simulink model "hw_interface_uart_data_sender"  (R2023b)
settings: Solver=FixedStepAuto  StartTime=0.0  StopTime=inf  FixedStep=0.001  RelTol=1e-3  EnableMultiTasking=on
undefined symbols (not defined in the file): LF
libraries: embeddedblockslib x1, mbedblockslib x1
settings Model: SimulationMode=external  ExtModeEnableFloating=off  ExtModeTrigDuration=10  Creator=kiraa  LastModifiedBy=kiraa
settings DataIOCC: SaveOutput=off  DSMLogging=off  SaveTime=off  TimeSaveName=time
settings OptimizationCC: StrengthReduction=on  PassReuseOutputArgsAs=Individual arguments  ZeroExternalMemoryAtStartup=off  ZeroInternalMemoryAtStartup=off  MaxStackSize=64  OptimizeBlockOrder=speed  OptimizationPriority=Speed  OptimizationCustomize=off  MultiThreadedLoops=on  EfficientTunableParamExpr=on
settings DebuggingCC: ParameterTunabilityLossMsg=error
settings HardwareCC: ProdBitPerPointer=32  ProdBitPerSizeT=32  ProdBitPerPtrDiffT=32  ProdLargestAtomicInteger=Long  ProdLargestAtomicFloat=Double  ProdWordSize=32  ProdLongLongMode=on  ProdHWDeviceType=ARM Compatible->ARM Cortex
settings SFSimCC: MATLABDynamicMemAlloc=off
settings RTWCC: Description=Embedded Coder  SystemTargetFile=ert.tlc  HardwareBoard=STM32 Nucleo F401RE  TemplateMakefile=ert_default_tmf  Toolchain=GNU Tools for ARM Embedded Processors
settings CodeAppCC: ForceParamTrailComments=on  IgnoreCustomStorageClasses=off  OperatorAnnotations=on  SimulinkDataObjDesc=on  SFDataObjDesc=on  InsertBlockDesc=on
settings ERTTargetCC: SupportContinuousTime=on  ExtMode=on  ExtModeTransport=3  ExtModeStaticAlloc=on  ExtModeStaticAllocSize=10000  ExtModeMexFile=ext_xcp  ExtModeMexArgs=1 3 115200  ExtModeIntrfLevel=Level2 - Open

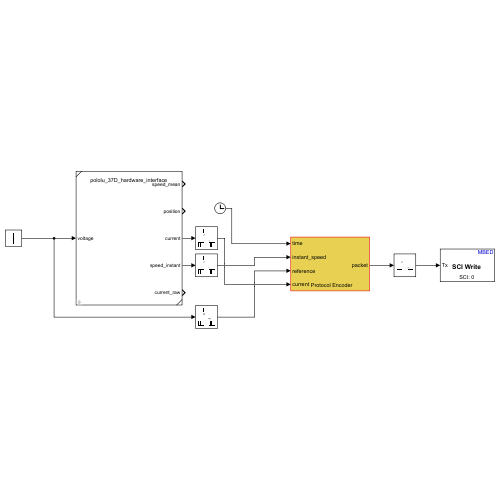
[thumbnail: Simulink's stored preview of the top-level diagram]
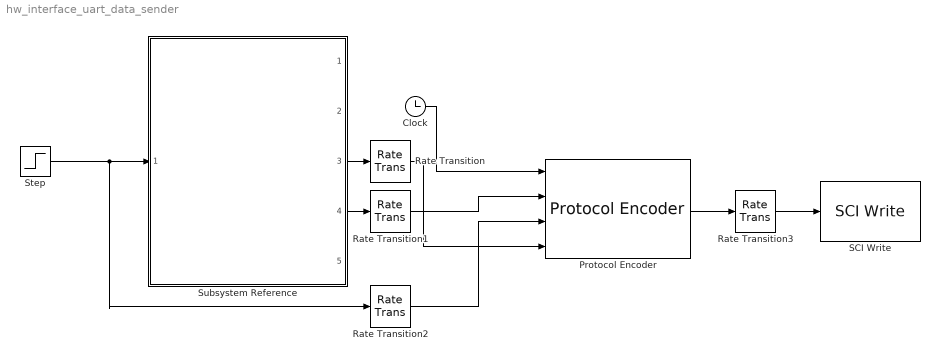
== system hw_interface_uart_data_sender ==
  Clock : Clock
  Protocol Encoder : embeddedblockslib/Protocol Encoder  Header='$'  FieldTable={ 'time', '1', 'double', 'Little endian'; 'instant_speed', '1', 'double', 'Little endian'; 'reference', '1', 'double', 'Little endian'; 'current', '1', 'double', 'Little endian' }  IsChecksumRequired=off  ChecksumAlgorithm=XOR of bytes  ChecksumSize=[]  TerminatorOption=LF ('\n')  CustomTerminatorVal=[]
      settings: LibrarySourceBlock=nucleoutilitieslib/Protocol Encoder
  Rate Transition{,1..3} (4 alike) : RateTransition
  SCI Write : mbedblockslib/SCI Write  SCIModule=0  Baudrate=uint32(9600)  Parity=None  StopBits=1  HardwareFlowControl=None  ByteOrder=LittleEndian  OutputStatus=off
      settings: LibrarySourceBlock=stmnucleorootlib/Common/SCI Write
  Step : Step  Time=2  After=0  SampleTime=0
  Subsystem Reference : Subsystem  ReferencedSubsystem=pololu_37D_hardware_interface  Ts=0.005  pwmFreq=2000
  wires:
  Step/1 -> Rate Transition2/1, Subsystem Reference/1
  Clock/1 -> Protocol Encoder/1
  Subsystem Reference/3 -> Rate Transition/1
  Subsystem Reference/4 -> Rate Transition1/1
  Rate Transition1/1 -> Protocol Encoder/2
  Rate Transition/1 -> Protocol Encoder/4
  Rate Transition2/1 -> Protocol Encoder/3
  Protocol Encoder/1 -> Rate Transition3/1
  Rate Transition3/1 -> SCI Write/1
